simulink model "Controladores_puzzle"  (R2024a)
settings: Solver=VariableStepAuto  StartTime=0.0  StopTime=60  RelTol=1e-3
libraries: slpidlib x2
settings Model: Creator=danii  LastModifiedBy=danii

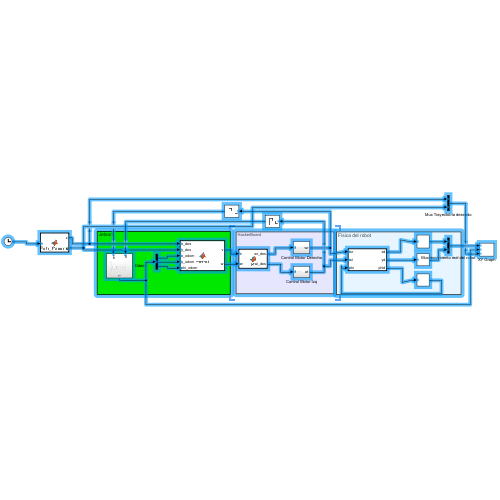
[thumbnail: Simulink's stored preview of the top-level diagram]
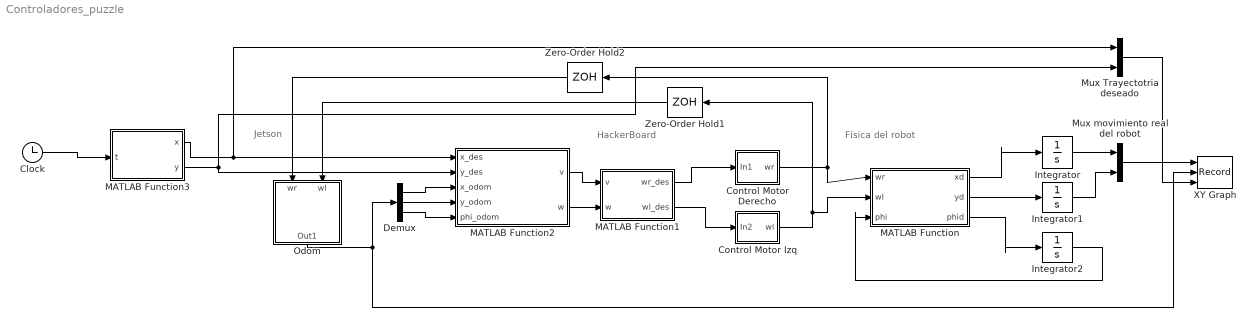
== system Controladores_puzzle ==
  note: Física del robot
  note: Jetson
  note: HackerBoard
  Clock : Clock
  Control Motor Derecho : Subsystem
  Control Motor Izq : Subsystem
  Demux : Demux  Outputs=3
  Integrator : Integrator  ContinuousStateAttributes='x'
  Integrator1 : Integrator  ContinuousStateAttributes='y'
  Integrator2 : Integrator  ContinuousStateAttributes='orientation'
  MATLAB Function : MATLAB Function  TreatAsAtomicUnit=on
  MATLAB Function1 : MATLAB Function  TreatAsAtomicUnit=on
  MATLAB Function2 : MATLAB Function  TreatAsAtomicUnit=on
  MATLAB Function3 : MATLAB Function  TreatAsAtomicUnit=on
  Mux Trayectotria deseado : Mux  Inputs=2
  Mux movimiento real del robot : Mux  Inputs=2
  Odom : Subsystem
  XY Graph : Record  FileSettingsInternal="{\"entries\":[{\"content\":{\"excelSettings\":{\"content\":{},\"type\":\"Streamout.ExcelSettings\"}},\"type\":\"Streamout.FileSettingStorage\",\"uuid\":\"\"}],\"packageUris\":[\"http:\\/\\/schema.mathworks.com\\/mf0\\/streamout_blocks\\/R2020a\"],\"version\":\"1.0\"}"  Layout=[1 1]  SignalsInternal="{\"entries\":[{\"content\":{\"signals\":[{\"content\":{\"blockPath\":[],\"dimensions\":[2],\"domain\":\"\",\"hasChildren\":true,\"lineColor\":\"#ff6929\",\"lineWidth\":2,\"port\":1,\"sid\":[\"\"],\"signalID\":1,\"signalName\":\"Mux movimiento real del robot\"},\"type\":\"RecordBlkView.Signal\",\"uuid\":\"\"},{\"content\":{\"blockPath\":[],\"channel\":[1],\"dimensions\":[2],\"domain\":\"\",\"lineColor\":\"#139fff\",\"parentID\":1,\"plots\":[ 1 ],\"port\":1,\"sid\":[\"\"],\"signalID\":2,\"signalName\":\"Mux movimiento real del robot\"},\"type\":\"RecordBlkView.Signal\",\"uuid\":\"\"},{\"content\":{\"blockPath\":[],\"dimensions\":[3],\"domain\":\"\",\"hasChildren\":true,\"lineColor\":\"#64d413\",\"lineWidth\":2,\"port\":2,\"sid\":[\"\"],\"signalID\":3,\"signalName\":\"Odom\"},\"type\":\"RecordBlkView.Signal\",\"uuid\":\"\"},{\"content\":{\"blockPath\":[],\"channel\":[1],\"dimensions\":[3],\"domain\":\"\",\"lineColor\":\"#b746ff\",\"parentID\":3,\"plots\":[ 1 ],\"port\":2,\"sid\":[\"\"],\"signalID\":4,\"signalName\":\"Odom\"},\"type\":\"RecordBlkView.Signal\",\"uuid\":\"\"},{\"content\":{\"blockPath\":[],\"dimensions\":[2],\"domain\":\"\",\"hasChildren\":true,\"lineColor\":\"#fe330a\",\"lineWidth\":2,\"port\":3,\"sid\":[\"\"],\"signalID\":5,\"signalName\":\"Mux Trayectotria deseado\"},\"type\":\"RecordBlkView.Signal\",\"uuid\":\"\"},{\"content\":{\"blockPath\":[],\"channel\":[1],\"dimensions\":[2],\"domain\":\"\",\"lineColor\":\"#fe330a\",\"lineWidth\":2,\"parentID\":5,\"plots\":[ 1 ],\"port\":3,\"sid\":[\"\"],\"signalID\":6,\"signalName\":\"Mux Trayectotria deseado\"},\"type\":\"RecordBlkView.Signal\",\"uuid\":\"\"},{\"content\":{\"blockPath\":[],\"channel\":[2],\"dimensions\":[2],\"domain\":\"\",\"lineColor\":\"#64d413\",\"parentID\":1,\"plots\":[ 1 ],\"port\":1,\"sid\":[\"\"],\"signalID\":7,\"signalName\":\"Mux movimiento real del robot\"},\"type\":\"RecordBlkView.Signal\",\"uuid\":\"\"},{\"content\":{\"blockPath\":[],\"channel\":[2],\"dimensions\":[3],\"domain\":\"\",\"lineColor\":\"#ff13a6\",\"parentID\":3,\"plots\":[ 1 ],\"port\":2,\"sid\":[\"\"],\"signalID\":8,\"signalName\":\"Odom\"},\"type\":\"RecordBlkView.Signal\",\"uuid\":\"\"},{\"content\":{\"blockPath\":[],\"channel\":[3],\"dimensions\":[3],\"domain\":\"\",\"lineColor\":\"#fe330a\",\"parentID\":3,\"port\":2,\"sid\":[\"\"],\"signalID\":9,\"signalName\":\"Odom\"},\"type\":\"RecordBlkView.Signal\",\"uuid\":\"\"},{\"content\":{\"blockPath\":[],\"channel\":[2],\"dimensions\":[2],\"domain\":\"\",\"lineColor\":\"#edb120\",\"lineWidth\":2,\"parentID\":5,\"plots\":[ 1 ],\"port\":3,\"sid\":[\"\"],\"signalID\":10,\"signalName\":\"Mux Trayectotria deseado\"},\"type\":\"RecordBlkView.Signal\",\"uuid\":\"\"}]},\"type\":\"RecordBlkView.InputSignals\",\"uuid\":\"\"}],\"packageUris\":[\"http:\\/\\/schema.mathworks.com\\/mf0\\/streamout_blocks\\/R2020a\"],\"version\":\"1.0\"}"  VisualizationBindings="{\"xyplotplugin\":{\"info\":[{\"series\":[{\"bindingParametersList\":[{\"parameter\":\"X-Axis\",\"signalID\":2,\"signalName\":\"Mux movimiento real del robot(1)\"},{\"parameter\":\"Y-Axis\",\"signalID\":7,\"signalName\":\"Mux movimiento real del robot(2)\"}],\"seriesID\":0},{\"bindingParametersList\":[{\"parameter\":\"X-Axis\",\"signalID\":4,\"signalName\":\"Odom(1)\"},{\"parameter\":\"Y-Axis\",\"signalID\":8,\"signalName\":\"Odom(2)\"}],\"seriesID\":1},{\"bindingParametersList\":[{\"parameter\":\"X-Axis\",\"signalID\":6,\"signalName\":\"Mux Trayectotria deseado(1)\"},{\"parameter\":\"Y-Axis\",\"signalID\":10,\"signalName\":\"Mux Trayectotria deseado(2)\"}],\"seriesID\":2}],\"subplotID\":1}]}}"  CompatibilityTag=XY
  Zero-Order Hold1 : ZeroOrderHold  SampleTime=0.01
  Zero-Order Hold2 : ZeroOrderHold  SampleTime=0.01
  wires:
  Zero-Order Hold2/1 -> Odom/1(wr)
  MATLAB Function3/2(y) -> Mux Trayectotria deseado/2, MATLAB Function2/2(y_des)
  Zero-Order Hold1/1 -> Odom/2(wl)
  MATLAB Function/3(phid) -> Integrator2/1
  Demux/1 -> MATLAB Function2/3(x_odom)
  Clock/1 -> MATLAB Function3/1(t)
  Integrator/1 -> Mux movimiento real del robot/1
  MATLAB Function3/1(x) -> Mux Trayectotria deseado/1, MATLAB Function2/1(x_des)
  Mux movimiento real del robot/1 -> XY Graph/1
  Demux/3 -> MATLAB Function2/5(phi_odom)
  MATLAB Function/1(xd) -> Integrator/1
  Odom/1(Out1) -> XY Graph/2, Demux/1
  Demux/2 -> MATLAB Function2/4(y_odom)
  MATLAB Function/2(yd) -> Integrator1/1
  Integrator1/1 -> Mux movimiento real del robot/2
  Control Motor Izq/1(wl) -> Zero-Order Hold1/1, MATLAB Function/2(wl)
  MATLAB Function1/2(wl_des) -> Control Motor Izq/1(In2)
  Control Motor Derecho/1(wr) -> MATLAB Function/1(wr), Zero-Order Hold2/1
  MATLAB Function2/2(w) -> MATLAB Function1/2(w)
  MATLAB Function1/1(wr_des) -> Control Motor Derecho/1(In1)
  Integrator2/1 -> MATLAB Function/3(phi)
  MATLAB Function2/1(v) -> MATLAB Function1/1(v)
  Mux Trayectotria deseado/1 -> XY Graph/3

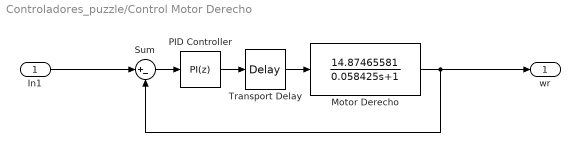
== system Controladores_puzzle/Control Motor Derecho ==
  In1 : Inport
  Motor Derecho : TransferFcn  Numerator=[14.87465581]  Denominator=[0.058425 1]
  PID Controller : slpidlib/PID Controller  Controller=PI  Form=Parallel  TimeDomain=Discrete-time  UseExternalTs=off  SampleTime=0.01  IntegratorMethod=Forward Euler  FilterMethod=Forward Euler  ControllerParametersSource=internal  P=0.03143  I=0.22281  UseKiTs=off  D=0  UseExternalDerivativeSource=off  N=100  UseFilter=on  TunerSelectOption=Transfer Function Based (PID Tuner App)  InitialConditionSource=internal  InitialConditionForIntegrator=0  InitialConditionForFilter=0  DifferentiatorICPrevScaledInput=0  ExternalReset=none  TrackingMode=off  Kt=1  LimitOutput=on  SatLimitsSource=internal  UpperSaturationLimit=1  LowerSaturationLimit=-1  LinearizeAsGain=on  AntiWindupMode=none  Kb=1  LimitIntegrator=off  UpperIntegratorSaturationLimit=inf  LowerIntegratorSaturationLimit=-inf  POutMin=[]  POutMax=[]  IOutMin=[]  IOutMax=[]  DOutMin=[]  DOutMax=[]  NOutMin=[]  NOutMax=[]  SumOutMin=[]  SumOutMax=[]  SaturationOutMin=[]  SaturationOutMax=[]  PParamMin=[]  PParamMax=[]  IParamMin=[]  IParamMax=[]  DParamMin=[]  DParamMax=[]  NParamMin=[]  NParamMax=[]  KbParamMin=[]  KbParamMax=[]  KtParamMin=[]  KtParamMax=[]  KbOutMin=[]  KbOutMax=[]  KtOutMin=[]  KtOutMax=[]  IntegratorOutMin=[]  IntegratorOutMax=[]  FilterOutMin=[]  FilterOutMax=[]  SumI1OutMin=[]  SumI1OutMax=[]  SumI2OutMin=[]  SumI2OutMax=[]  SumI3OutMin=[]  SumI3OutMax=[]  SumI4OutMin=[]  SumI4OutMax=[]  SumDOutMin=[]  SumDOutMax=[]  DifferentiatorOutMin=[]  DifferentiatorOutMax=[]  FilterDiffOutCoefMin=[]  FilterDiffOutCoefMax=[]  ReciprocalOutMin=[]  ReciprocalOutMax=[]  SumDenOutMin=[]  SumDenOutMax=[]  SumNumOutMin=[]  SumNumOutMax=[]  DivideOutMin=[]  DivideOutMax=[]  UdiffTsProdOutMin=[]  UdiffTsProdOutMax=[]  NTsProdOutMin=[]  NTsProdOutMax=[]  UintegralTsProdOutMin=[]  UintegralTsProdOutMax=[]  UngainTsProdOutMin=[]  UngainTsProdOutMax=[]  ClampingZeroOutDataTypeStr=Inherit: Inherit via back propagation  ClampingZeroOutMin=[]  ClampingZeroOutMax=[]  FilterDenConstantOutDataTypeStr=Inherit: Inherit via back propagation  FilterDenConstantOutMin=[]  FilterDenConstantOutMax=[]  PCopyOutDataTypeStr=Inherit: Inherit via back propagation  PCopyOutMin=[]  PCopyOutMax=[]  NCopyOutDataTypeStr=Inherit: Inherit via back propagation  NCopyOutMin=[]  NCopyOutMax=[]  IntegratorContinuousStateAttributes=''  IntegratorStateMustResolveToSignalObject=off  IntegratorRTWStateStorageClass=Auto  FilterContinuousStateAttributes=''  FilterStateMustResolveToSignalObject=off  FilterRTWStateStorageClass=Auto  ParallelPVariant=InternalParameters  IdealPVariant=Disabled  IVariant=InternalParameters  DVariant=Disabled  IntegratorVariant=Discrete  SatVariant=Enabled  AWVariant=Passthrough  PCopyVariant=Disabled  TRVariant=Disabled  FdbkBlocksVariant=Forward  IdealPFdbkVariant=Disabled  SatFdbkVariant=Disabled  DerivativeFilterVariant=Disabled  NVariant=Disabled  NCopyVariant=Disabled_SignalSpec  FilterICVariant=Disabled  IntegratorICVariant=InternalICs  ExternalResetVariant=Disabled  TRSumVariant=Passthrough  SumFdbkVariant=Disabled  SumVariant=Sum_PI  TsampFilterVariant=InternalTs  TsampNgainVariant=Passthrough  TsampIntegralVariant=Disabled_SignalSpec  ExternalSaturationOutDataTypeStr=Inherit: Same as second input  DerivativeSourceVariant=Disabled
  Sum : Sum  Inputs=|+-
  Transport Delay : TransportDelay  DelayTime=0.043735
  wr : Outport
  wires:
  PID Controller/1 -> Transport Delay/1
  Transport Delay/1 -> Motor Derecho/1
  In1/1 -> Sum/1
  Motor Derecho/1 -> wr/1, Sum/2
  Sum/1 -> PID Controller/1

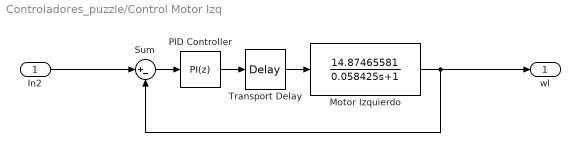
== system Controladores_puzzle/Control Motor Izq ==
  In2 : Inport
  Motor Izquierdo : TransferFcn  Numerator=[14.87465581]  Denominator=[0.058425 1]
  PID Controller : slpidlib/PID Controller  Controller=PI  Form=Parallel  TimeDomain=Discrete-time  UseExternalTs=off  SampleTime=0.01  IntegratorMethod=Forward Euler  FilterMethod=Forward Euler  ControllerParametersSource=internal  P=0.03143  I=0.22281  UseKiTs=off  D=0  UseExternalDerivativeSource=off  N=100  UseFilter=on  TunerSelectOption=Transfer Function Based (PID Tuner App)  InitialConditionSource=internal  InitialConditionForIntegrator=0  InitialConditionForFilter=0  DifferentiatorICPrevScaledInput=0  ExternalReset=none  TrackingMode=off  Kt=1  LimitOutput=on  SatLimitsSource=internal  UpperSaturationLimit=1  LowerSaturationLimit=-1  LinearizeAsGain=on  AntiWindupMode=none  Kb=1  LimitIntegrator=off  UpperIntegratorSaturationLimit=inf  LowerIntegratorSaturationLimit=-inf  POutMin=[]  POutMax=[]  IOutMin=[]  IOutMax=[]  DOutMin=[]  DOutMax=[]  NOutMin=[]  NOutMax=[]  SumOutMin=[]  SumOutMax=[]  SaturationOutMin=[]  SaturationOutMax=[]  PParamMin=[]  PParamMax=[]  IParamMin=[]  IParamMax=[]  DParamMin=[]  DParamMax=[]  NParamMin=[]  NParamMax=[]  KbParamMin=[]  KbParamMax=[]  KtParamMin=[]  KtParamMax=[]  KbOutMin=[]  KbOutMax=[]  KtOutMin=[]  KtOutMax=[]  IntegratorOutMin=[]  IntegratorOutMax=[]  FilterOutMin=[]  FilterOutMax=[]  SumI1OutMin=[]  SumI1OutMax=[]  SumI2OutMin=[]  SumI2OutMax=[]  SumI3OutMin=[]  SumI3OutMax=[]  SumI4OutMin=[]  SumI4OutMax=[]  SumDOutMin=[]  SumDOutMax=[]  DifferentiatorOutMin=[]  DifferentiatorOutMax=[]  FilterDiffOutCoefMin=[]  FilterDiffOutCoefMax=[]  ReciprocalOutMin=[]  ReciprocalOutMax=[]  SumDenOutMin=[]  SumDenOutMax=[]  SumNumOutMin=[]  SumNumOutMax=[]  DivideOutMin=[]  DivideOutMax=[]  UdiffTsProdOutMin=[]  UdiffTsProdOutMax=[]  NTsProdOutMin=[]  NTsProdOutMax=[]  UintegralTsProdOutMin=[]  UintegralTsProdOutMax=[]  UngainTsProdOutMin=[]  UngainTsProdOutMax=[]  ClampingZeroOutDataTypeStr=Inherit: Inherit via back propagation  ClampingZeroOutMin=[]  ClampingZeroOutMax=[]  FilterDenConstantOutDataTypeStr=Inherit: Inherit via back propagation  FilterDenConstantOutMin=[]  FilterDenConstantOutMax=[]  PCopyOutDataTypeStr=Inherit: Inherit via back propagation  PCopyOutMin=[]  PCopyOutMax=[]  NCopyOutDataTypeStr=Inherit: Inherit via back propagation  NCopyOutMin=[]  NCopyOutMax=[]  IntegratorContinuousStateAttributes=''  IntegratorStateMustResolveToSignalObject=off  IntegratorRTWStateStorageClass=Auto  FilterContinuousStateAttributes=''  FilterStateMustResolveToSignalObject=off  FilterRTWStateStorageClass=Auto  ParallelPVariant=InternalParameters  IdealPVariant=Disabled  IVariant=InternalParameters  DVariant=Disabled  IntegratorVariant=Discrete  SatVariant=Enabled  AWVariant=Passthrough  PCopyVariant=Disabled  TRVariant=Disabled  FdbkBlocksVariant=Forward  IdealPFdbkVariant=Disabled  SatFdbkVariant=Disabled  DerivativeFilterVariant=Disabled  NVariant=Disabled  NCopyVariant=Disabled_SignalSpec  FilterICVariant=Disabled  IntegratorICVariant=InternalICs  ExternalResetVariant=Disabled  TRSumVariant=Passthrough  SumFdbkVariant=Disabled  SumVariant=Sum_PI  TsampFilterVariant=InternalTs  TsampNgainVariant=Passthrough  TsampIntegralVariant=Disabled_SignalSpec  ExternalSaturationOutDataTypeStr=Inherit: Same as second input  DerivativeSourceVariant=Disabled
  Sum : Sum  Inputs=|+-
  Transport Delay : TransportDelay  DelayTime=0.043735
  wl : Outport
  wires:
  PID Controller/1 -> Transport Delay/1
  Sum/1 -> PID Controller/1
  Motor Izquierdo/1 -> wl/1, Sum/2
  In2/1 -> Sum/1
  Transport Delay/1 -> Motor Izquierdo/1

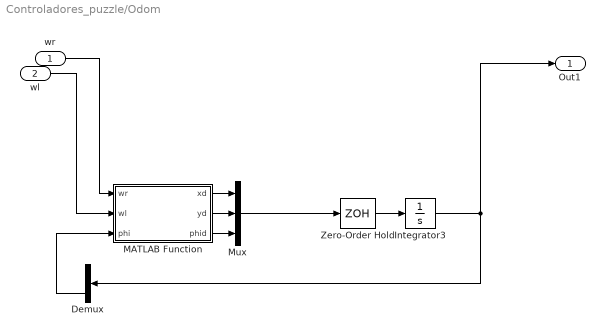
== system Controladores_puzzle/Odom ==
  wr : Inport
  wl : Inport  Port=2
  Demux : Demux  Outputs=3
  Integrator3 : Integrator  InitialCondition=[0,0,0]
  MATLAB Function : MATLAB Function  TreatAsAtomicUnit=on
  Mux : Mux  Inputs=3
  Zero-Order Hold : ZeroOrderHold  SampleTime=0.01
  Out1 : Outport
  wires:
  Mux/1 -> Zero-Order Hold/1
  wl/1 -> MATLAB Function/2(wl)
  Integrator3/1 -> Demux/1, Out1/1
  Zero-Order Hold/1 -> Integrator3/1
  wr/1 -> MATLAB Function/1(wr)
  MATLAB Function/1(xd) -> Mux/1
  MATLAB Function/2(yd) -> Mux/2
  MATLAB Function/3(phid) -> Mux/3
  Demux/3 -> MATLAB Function/3(phi)

== matlab function Controladores_puzzle/MATLAB Function1 ==
  data: v input; wr_des output; w input; wl_des output
function [wr_des,wl_des] = IK(v,w) %Twist local

R=0.0505;
b=0.1712;

wr_des=(v/R)+(w*b/(2*R));
wl_des=(v/R)-(w*b/(2*R));

== matlab function Controladores_puzzle/MATLAB Function ==
  data: wr input; xd output; wl input; phi input; yd output; phid output
function [xd, yd, phid] = ROBOT(wr,wl,phi) %Psi es el heading.
% El heading es la orientación (dirección del mov)
% Las letras latina son translacionales, las letras griegas son
% rotacionales)
%El sufijo d significa (derivada) (Lo transforma en velocidad)

R=0.0505;%Metros
b=0.1712; %Metros

xd= (wr+wl)*(R/2)*cos(phi); %Vxl*Cos(phi)
yd= (wr+wl)*(R/2)*sin(phi); %Vxl*Sin(phi)
phid=(wr-wl)*(R/b);

== matlab function Controladores_puzzle/MATLAB Function2 ==
  data: x_des input; y_des input; x_odom input; v output; y_odom input; phi_odom input; w output
function [v, w] = control(x_des, y_des, x_odom, y_odom, phi_odom)
    % Ganancias
    Kl = 1;     % 1/s
    Kw = 1.52;  % rad/s

    mode='turn_then_go'; %Modificar para cambiar el tipo de control
    %mode='turn_while_go';
    %mode='carrot_chasing';
    %mode = 'lyapunov';



    % Errores
    e_pos = sqrt((x_des - x_odom)^2 + (y_des - y_odom)^2);
    phi_des = atan2(y_des - y_odom, x_des - x_odom);
    e_ori = phi_des - phi_odom;
    e_ori = atan2(sin(e_ori), cos(e_ori));

    switch mode
        case 'turn_while_go'  % Turn and go simultaneously
            if abs(e_ori) > 1 || e_pos < 0.01
                e_pos = 0;
            end

            if abs(e_ori) < 1 * pi / 180
                e_ori = 0;
            end

            v = max(min(e_pos * Kl, 0.2), -0.2);
            w = max(min(e_ori * Kw, 0.2), -0.2);

        case 'turn_then_go'  % Turn first, then go
            angle_threshold = 5 * pi / 180;  % 5 degrees

            if abs(e_ori) > angle_threshold
                v = 0;  % no forward motion
                w = max(min(e_ori * Kw, 0.2), -0.2);  % turn to desired orientation
            elseif e_pos > 0.01
                w = 0;  % orientation is okay, move forward
                v = max(min(e_pos * Kl, 0.2),-0.2);
            else
                v = 0;
                w = 0;  % goal reached
            end
        
        case 'lyapunov'
          
            v_ri = 0.2;    % velocidad de referencia (m/s)
            k1   = 0.025;    % coeficiente k1 > 0
            k2   = 0.01;    % coeficiente k2 > 0
        
         
            dx = x_des - x_odom;
            dy = y_des - y_odom;
            rho = sqrt(dx^2 + dy^2);      % distancia al objetivo
        
       
            theta_G  = atan2(dy, dx);                              
            theta_er = atan2(sin(theta_G - phi_odom), cos(theta_G - phi_odom));  
             
        
           
            v = v_ri * cos(theta_er);
        
            %  ω = k1*θ_er + [ v_ri cos(θ_er) sin(θ_er) (θ_er + k2*θ_G ) ] / θ_er
            if abs(theta_er) > 1e-6
                w = k1 * theta_er + ...
                    ( v_ri * cos(theta_er) * sin(theta_er) * ( theta_er + k2 * theta_G ) ) ...
                    / theta_er;
            else
                % caso θ_er ≈ 0 → ≈ k1·θ_er
                w = k1 * theta_er;
            end

            v = max(min(v, 0.2), -0.2);   % límite en v
            w = max(min(w, 0.6), -0.6);   % límite en ω
        
            if rho < 0.02
                v = 0;
                w = 0;
            end

        case 'carrot_chasing'
            L = 0.5;  % distancia de anticipación
            dx = x_des - x_odom;
            dy = y_des - y_odom;
            d_total = sqrt(dx^2 + dy^2);
        
            if d_total < 0.05  % umbral para detener
                v = 0;
                w = 0;
                return;
            end
        
            % Calcular el punto carrot
            if d_total > L
                x_carrot = x_odom + L * dx / d_total;
                y_carrot = y_odom + L * dy / d_total;
            else
                x_carrot = x_des;
                y_carrot = y_des;
            end
        
            phi_carrot = atan2(y_carrot - y_odom, x_carrot - x_odom);
            e_phi = atan2(sin(phi_carrot - phi_odom), cos(phi_carrot - phi_odom));
        
            v = max(min(Kl * d_total, 0.2),-0.2);
            w = max(min(Kw * e_phi, 0.2), -0.2);

        otherwise
            error('Verifica el nombre del controlador.');
    end
end

== matlab function Controladores_puzzle/Odom/MATLAB Function ==
  data: wr input; xd output; wl input; phi input; yd output; phid output
function [xd, yd, phid] = cinematica(wr,wl,phi) %Psi es el heading.
% El heading es la orientación (dirección del mov)
% Las letras latina son translacionales, las letras griegas son
% rotacionales)
%El sufijo d significa (derivada) (Lo transforma en velocidad)

R=0.0505;%Metros
b=0.1712; %Metros

xd= (wr+wl)*(R/2)*cos(phi); %Vxl*Cos(phi)
yd= (wr+wl)*(R/2)*sin(phi); %Vxl*Sin(phi)
phid=(wr-wl)*(R/b);

== matlab function Controladores_puzzle/MATLAB Function3 ==
  data: x output; t input; y output
function [x,y] = Path_Planning(t)

radio=1;
w=(0.1/radio);

%if t < 60
%        x = 2;
%        y = 0;
%elseif t<120
        % Punto nuevo después de 65 segundos
%        x = 2;   
%        y = 2;  
%elseif t<180
%        x = 0;   
%        y = 2;
%else
%    x = 0;   
%    y = 0;

%end
x=radio*sin(w*t);
y=-radio*cos(w*t)+radio;
%x=-1;
%y=-1;
